simulink model "untitled"  (R2025a)
settings: Solver=VariableStepAuto  StartTime=0.0  StopTime=10.0  RelTol=1e-3
settings Model: Creator=nikul  LastModifiedBy=nikul

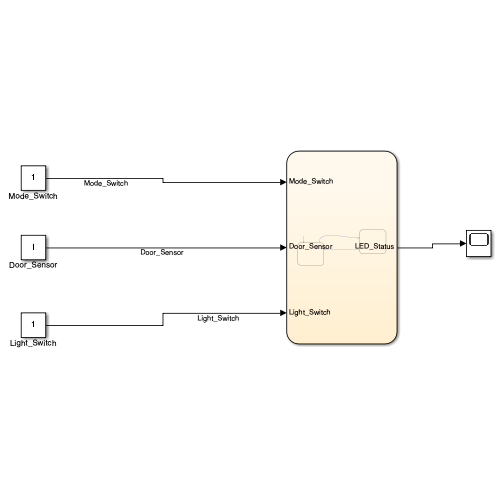
[thumbnail: Simulink's stored preview of the top-level diagram]
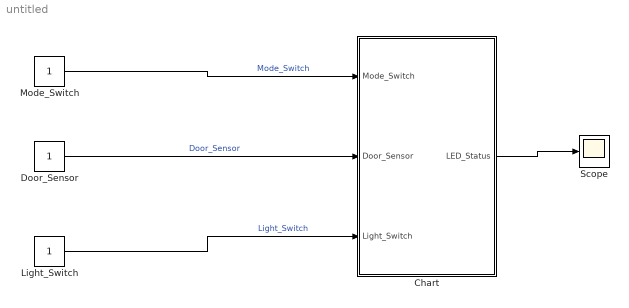
== system untitled ==
  Chart : Stateflow chart  TreatAsAtomicUnit=on
  Door_Sensor : Constant
  Light_Switch : Constant
  Mode_Switch : Constant
  Scope : Scope
  wires:
  Mode_Switch/1 -> Chart/1(Mode_Switch)  "Mode_Switch"
  Door_Sensor/1 -> Chart/2(Door_Sensor)  "Door_Sensor"
  Light_Switch/1 -> Chart/3(Light_Switch)  "Light_Switch"
  Chart/1(LED_Status) -> Scope/1

== stateflow chart untitled/Chart ==
  state Manual_Mode
    during:
    if (Light_Switch == 1)
    LED_Status = 1;
    else
    LED_Status = 0;
    end
  state Auto_Mode
    during:
    if (Door_Sensor == 1)
    LED_Status = 1;
    else
    LED_Status = 0;
    end
  Auto_Mode -> Manual_Mode : [Mode_Switch == 1]
  (default) -> Auto_Mode
  Manual_Mode -> Auto_Mode : [Mode_Switch == 0]
  data: Mode_Switch input; Door_Sensor input; Light_Switch input; LED_Status output
